simulink model "gravCompTesting"  (Simulink 8.0)
settings: Solver=FixedStepDiscrete  StartTime=0.0  StopTime=inf  FixedStep=Ts  RelTol=1e-3
values from neighbouring files (symbols this model uses):
  ROBOT_DOF = 20    [init_jointTorqController_reachPos.m]
libraries: WBToolboxLibrary x6
settings Model: Creator=nunoguedelha  LastModifiedBy=nunoguedelha

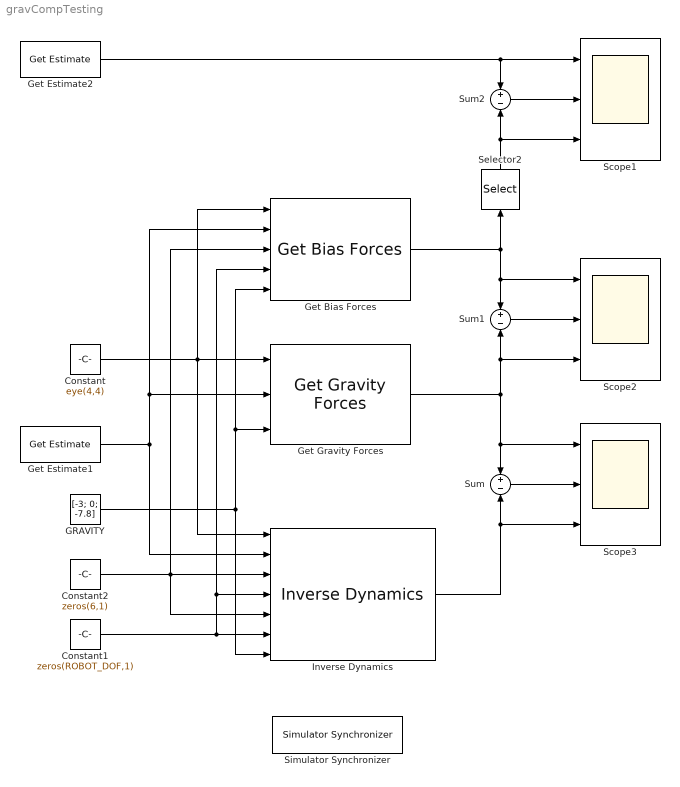
== system gravCompTesting ==
  Constant : Constant  Value=eye(4,4)  VectorParams1D=off  SampleTime=-1
  Constant1 : Constant  Value=zeros(ROBOT_DOF,1)  SampleTime=-1
  Constant2 : Constant  Value=zeros(6,1)  SampleTime=-1
  GRAVITY : Constant  Value=[-3; 0; -7.8]  SampleTime=-1
  Get Bias Forces : WBToolboxLibrary/wholeBodyModel/Dynamics/Get Bias Forces  robotName=WBT_robotName  localName=WBT_modelName  wbiFile=WBT_wbiFilename  wbiList=WBT_wbiList  explicitGravity=on
  Get Estimate1 : WBToolboxLibrary/wholeBodyStates/Get Estimate  estimateType=Joints Position  robotName=WBT_robotName  localName=WBT_modelName  wbiFile=WBT_wbiFilename  wbiList=WBT_wbiList
  Get Estimate2 : WBToolboxLibrary/wholeBodyStates/Get Estimate  estimateType=Joints Torque  robotName=WBT_robotName  localName=WBT_modelName  wbiFile=WBT_wbiFilename  wbiList=WBT_wbiList
  Get Gravity Forces : WBToolboxLibrary/wholeBodyModel/Dynamics/Get Gravity Forces  robotName=WBT_robotName  localName=WBT_modelName  wbiFile=WBT_wbiFilename  wbiList=WBT_wbiList  explicitGravity=on
  Inverse Dynamics : WBToolboxLibrary/wholeBodyModel/Dynamics/Inverse Dynamics  robotName=WBT_robotName  localName=WBT_modelName  wbiFile=WBT_wbiFilename  wbiList=WBT_wbiList  explicitGravity=on
  Scope1 : Scope  NumInputPorts=3
      settings: YMin=-2.5~-0.09~-2.5  YMax=1.25~0.06~1.25
  Scope2 : Scope  NumInputPorts=3
      settings: YMin=-25~-1~-25  YMax=250~1~250
  Scope3 : Scope  NumInputPorts=3
      settings: YMin=-25~-1~-25  YMax=300~1~300  SaveName=ScopeData2
  Selector2 : Selector  InputPortWidth=6+ROBOT_DOF  IndexOptions=Index vector (dialog)  Indices=[7:26]  OutputSizes=1
  Simulator Synchronizer : WBToolboxLibrary/Utilities/Simulator Synchronizer  period=0.01  serverPortName='/clock/rpc'  clientPortName='/WBT_synchronizer/rpc:o'
  Sum : Sum  Inputs=+|-
  Sum1 : Sum  Inputs=+|-
  Sum2 : Sum  Inputs=+|-
  wires:
  Constant/1 -> Get Bias Forces/1, Inverse Dynamics/1, Get Gravity Forces/1
  Get Estimate1/1 -> Inverse Dynamics/2, Get Bias Forces/2, Get Gravity Forces/2
  Constant1/1 -> Inverse Dynamics/6, Get Bias Forces/4, Inverse Dynamics/4
  Inverse Dynamics/1 -> Scope3/3, Sum/2
  Sum/1 -> Scope3/2
  Get Estimate2/1 -> Scope1/1, Sum2/1
  Sum2/1 -> Scope1/2
  GRAVITY/1 -> Get Bias Forces/5, Get Gravity Forces/3, Inverse Dynamics/7
  Get Bias Forces/1 -> Selector2/1, Scope2/1, Sum1/1
  Sum1/1 -> Scope2/2
  Get Gravity Forces/1 -> Scope2/3, Sum1/2, Scope3/1, Sum/1
  Selector2/1 -> Scope1/3, Sum2/2
  Constant2/1 -> Get Bias Forces/3, Inverse Dynamics/5, Inverse Dynamics/3
